simulink model "new_model_like_me"  (R2023a)
settings: Solver=FixedStepDiscrete  StartTime=0.0  StopTime=5  FixedStep=Ts  RelTol=1e-3  EnableMultiTasking=on
PreLoadFcn:
  | parameters_for_model_inn;
StopFcn:
  | ee_addSimlogTimeStamp(bdroot)
values from neighbouring files (symbols this model uses):
  deg = 10    [parameters_for_model_inn.m]
  Jm = 0.001368    [parameters_for_model_inn.m]
  Kaw_omega = 1    [parameters_for_model_inn.m]
  Ki_id = 3    [parameters_for_model_inn.m]
  Ki_iq = 20    [parameters_for_model_inn.m]
  Ki_omega = 2.2    [parameters_for_model_inn.m]
  Kp_id = 0.01    [parameters_for_model_inn.m]
  Kp_iq = 1.8    [parameters_for_model_inn.m]
  Kp_omega = 0.6    [parameters_for_model_inn.m]
  Kp_pos = 0.8    [parameters_for_model_inn.m]
  Ld = 0.00595    [parameters_for_model_inn.m]
  LimA2down = -80    [parameters_for_model_inn.m]
  LimA2up = 64    [parameters_for_model_inn.m]
  Lq = 0.00595    [parameters_for_model_inn.m]
  p = 4    [parameters_for_model_inn.m]
  psim = 0.180694733685904    (= 0.180694733686)    [parameters_for_model_inn.m]
  Red = 34.68    [parameters_for_model_inn.m]
  Tid_start = Tiq_stop + 0.02    (= 0.1)    [parameters_for_model_inn.m]
  Tid_stop = Tid_start + 0.04    (= 0.14)    [parameters_for_model_inn.m]
  Tiq_start = 0.02    [parameters_for_model_inn.m]
  Tiq_stop = Tiq_start + 0.06    (= 0.08)    [parameters_for_model_inn.m]
  Tomega_start = Tid_stop + 0.02    (= 0.16)    [parameters_for_model_inn.m]
  Tomega_stop = Tomega_start + 0.06    (= 0.22)    [parameters_for_model_inn.m]
  Tpos_start = Tomega_stop + 0.02    (= 0.24)    [parameters_for_model_inn.m]
  Tpos_stop = Tpos_start + 0.06    (= 0.3)    [parameters_for_model_inn.m]
  Ts = 5e-5    (= 5e-05)    [parameters_for_model_inn.m]
  Tsi = Ts * 20    (= 0.001)    [parameters_for_model_inn.m]
  Tso = Ts * 200    (= 0.01)    [parameters_for_model_inn.m]
  V1 = 250    [parameters_for_model_inn.m]
  Vnom = 300    [parameters_for_model_inn.m]
  Wmax = 7000    [parameters_for_model_inn.m]
  Wnom = 1800    [parameters_for_model_inn.m]
undefined symbols (not defined in the file or in its folder): DiscIntNeverNeededParam, Kd_pos, Ki_pos, Kn_pos, Tpos, X, Y, Z
libraries: nesl_utility x18, fl_lib x10, sm_lib x8, slctrlblks x6, ee_lib x5, eeTransforms x3, dspfdesign x3, eePmsmCurrentController x2, simulink x2, slpidlib x2, robotmaniplib x2, batteryecm_lib x1
(part 1 of 2)
CloseFcn:
  | try,close(h1_ee_ipmsm_velocity_control),end
  | clear h1_ee_ipmsm_velocity_control
  | 
  | clear simlog_ee_ipmsm_velocity_control
  | clear logsout_ee_ipmsm_velocity_control
  | 
  | clear Pmax Tmax p psim Ld Lq L0 Rs Jm Imax Wmax ans RT_Time RedTrq Red
  | clear Cdc Vnom V1 AH0
  | clear Ts fsw Tpos Tsi Tso Kp_id Ki_id Kp_iq Ki_iq Clock_fcn fn
  | clear numd_id dend_id numd_iq dend_iq psim
  | clear Kp_omega Ki_omega Kn_omega numd_omega dend_omega Kp_pos Ki_pos Kn_pos Kd_pos
  | clear ID_MAP IQ_MAP RPM_VECT TQ_VECT VDC_VECT
  | clear Link2 ArmInfo tout
Description:
  | IPMSM Full Control
settings Model: PauseTimes=0  Creator=KolobovBK  LastModifiedBy=kolobov_bk
settings SolverCC: AlgebraicLoopSolver=TrustRegion  AutoInsertRateTranBlk=on  MaxZcPerStep=1
settings DataIOCC: MaxDataPoints=210000  DSMLogging=off  ReturnWorkspaceOutputs=off  SignalLoggingName=logsout_ee_ipmsm_velocity_control
settings OptimizationCC: ReuseModelBlockBuffer=off  LifeSpan=inf
settings DebuggingCC: UnderspecifiedInitializationDetection=Classic  MergeDetectMultiDrivingBlocksExec=none  UnconnectedInputMsg=warning  UnconnectedOutputMsg=warning  UnconnectedLineMsg=warning  SFUnexpectedBacktrackingDiag=warning  SFNoUnconditionalDefaultTransitionDiag=warning  SFExecutionAtInitializationDiag=none  ArithmeticOperatorsInVariantConditions=warning
settings ModelReferenceCC: EnableRefExpFcnMdlSchedulingChecks=on
settings SFSimCC: SimUseLocalCustomCode=off  CustomCodeUndefinedFunction=UseInterfaceOnly
settings RTWCC: RTWUseLocalCustomCode=off  DLArmComputeVersion=19.05
settings CodeAppCC: StateflowObjectComments=on
settings GRTTargetCC: TargetLangStandard=C89/C90 (ANSI)
settings ConfigComp: CovMetricSettings=dw  CovSaveCumulativeToWorkspaceVar=on  CovSaveSingleToWorkspaceVar=on  CovExternalEMLEnable=off
settings SimscapeCC: SimscapeNormalizeSystem=off  SimscapeLogType=all  SimscapeLogSimulationStatistics=on  SimscapeLogName=simlog_ee_ipmsm_velocity_control  SimscapeLogDataHistory=210000

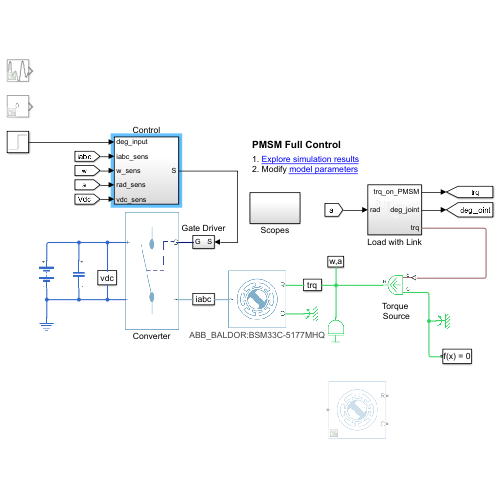
[thumbnail: Simulink's stored preview of the top-level diagram]
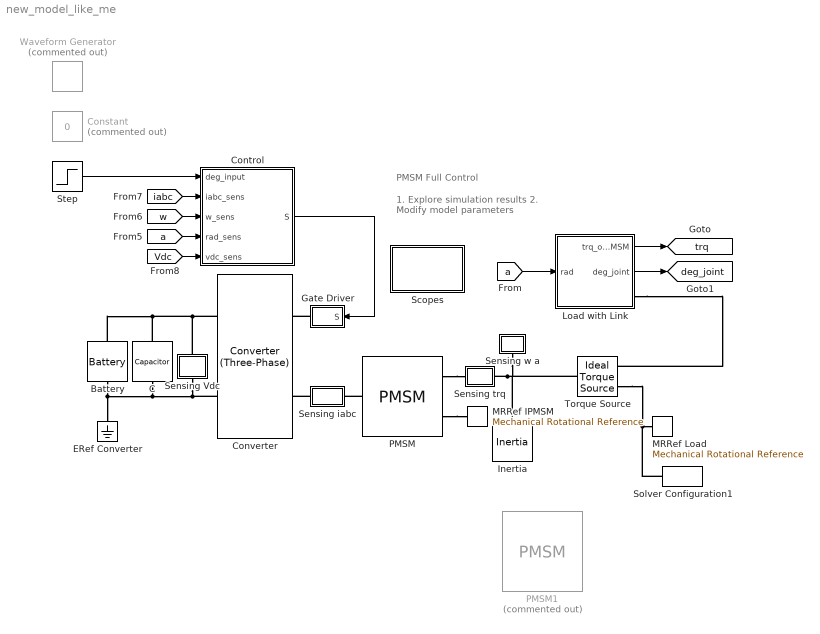
== system new_model_like_me ==
  note: PMSM Full Control
  note: 1. Explore simulation results
      | 2. Modify model parameters
  Battery : batteryecm_lib/Battery  Vnom=Vnom V  prm_dir=1  R1_dis=2 Ohm  R1_ch=2 Ohm  R1=0.001 Ohm  prm_AH=1  AH=300 hr*A  V1=V1 V  AH1=100 hr*A  prm_R2=1  R2=2000 Ohm  Tmeas=298.15 K  charge_measurement_port=simscape.enum.battery.enable.no  prm_dyn=1  Rp1=0.005 Ohm  tau1=30 s  Rp2=0.005 Ohm  tau2=30 s  Rp3=0.005 Ohm  tau3=30 s  Rp4=0.005 Ohm  tau4=30 s  Rp5=0.005 Ohm  tau5=30 s  prm_fade=1  N_fade=100  AH_fade=45 hr*A  R1_fade=2.02 Ohm  R1_ch_fade=2.02 Ohm  V1_fade=10.35 V  prm_age=1  prm_age_OCV=1  OCV_age=0.9  SOC_age=60  Tmeas_age=298.15 K  delta_time_age_vec=[0] d  temperature_age_vec=[273] K  OCV_scaling_age=2.2134e6  OCV_offset_age=1.632e6  temp_exp_age=0.515833569 V  t_exp_age=0.75  Vnom_T2=12 V  R1_T2=2.2 Ohm  R1_T2_dis=2.2 Ohm  R1_T2_ch=2.2 Ohm  V1_T2=11.4 V  R2_T2=2200 Ohm  Rp1_T2=0.005 Ohm  tau1_T2=30 s  Rp2_T2=0.005 Ohm  tau2_T2=30 s  Rp3_T2=0.005 Ohm  tau3_T2=30 s  Rp4_T2=0.005 Ohm  tau4_T2=30 s  Rp5_T2=0.005 Ohm  tau5_T2=30 s  Tmeas2=273.15 K  thermal_port=simscape.enum.thermaleffects.omit  thermal_mass=30000 J/K  i_specify=off  i_priority=None  i=0 A  i_nominal_specify=off  i_nominal_unit=A  i_nominal_value=1  v_specify=on  v_priority=High  v=300 V  v_nominal_specify=off  v_nominal_unit=V  v_nominal_value=1  charge_specify=on  charge_priority=High  charge=AH0 hr*A  charge_nominal_specify=off  charge_nominal_unit=A*hr  charge_nominal_value=1  num_cycles_specify=off  num_cycles_priority=High  num_cycles=0  num_cycles_nominal_specify=off  num_cycles_nominal_unit=1  num_cycles_nominal_value=1  temperature_specify=off  temperature_priority=High  temperature=298.15 K  temperature_nominal_specify=off  temperature_nominal_unit=K  temperature_nominal_value=1
  C : fl_lib/Electrical/Electrical Elements/Capacitor  c=Cdc F  r=1e-6 Ohm  g=0 1/Ohm  i_specify=off  i_priority=None  i=0 A  i_nominal_specify=off  i_nominal_unit=A  i_nominal_value=1  v_specify=off  v_priority=None  v=0 V  v_nominal_specify=off  v_nominal_unit=V  v_nominal_value=1  vc_specify=on  vc_priority=None  vc=Vnom V  vc_nominal_specify=off  vc_nominal_unit=V  vc_nominal_value=1
  Constant : Constant  Commented=on  Value=0
  Control : Subsystem
  Converter : ee_lib/Semiconductors & Converters/Converters/Converter (Three-Phase)  port_option=ee.enum.threePhasePort.composite  device_type=3  K=0  Vf=0.8 V  Ron=0.001 Ohm  Rds=0.001 Ohm  Goff=1e-5 1/Ohm  Vgt=1 V  Vgt_off=-1 V  Ih=1 A  Vth=0.5 V  diode_param=2  diode_Vf=0.8 V  diode_Ron=0.001 Ohm  diode_Goff=1e-5 1/Ohm  diode_C=50 nF  diode_iRM=-235 A  diode_iF=300 A  diode_idot=-50 A/us  diode_trr_param=1  diode_trr_factor=3  diode_trr=15 us  diode_Qrr=1.5e+3 s*uA  snubber_type=0  Cs=1e-7 F  Rs=0.1 Ohm
  ERef Converter : fl_lib/Electrical/Electrical Elements/Electrical Reference
  Gate Driver : Subsystem
  Inertia : fl_lib/Mechanical/Rotational Elements/Inertia  inertia=Jm kg*m^2  num_ports=foundation.enum.numPorts2.one  w_specify=on  w_priority=High  w=0 rpm  w_nominal_specify=off  w_nominal_unit=rad/s  w_nominal_value=1  t_specify=off  t_priority=High  t=0 N*m  t_nominal_specify=off  t_nominal_unit=N*m  t_nominal_value=1
  Load with Link : Subsystem
  MRRef IPMSM : fl_lib/Mechanical/Rotational Elements/Mechanical Rotational Reference
  MRRef Load : fl_lib/Mechanical/Rotational Elements/Mechanical Rotational Reference
  PMSM : ee_lib/Electromechanical/Permanent Magnet/PMSM  Tag={'toolbox/physmod/elec/library/m/ee_lib_parts';'Electromechanical/Permanent_Magnet/PMSM/ABB_BALDOR/BSM33C_5177MHQ.xml'}  port_option=ee.enum.threePhasePort.composite  winding_type=ee.enum.statorconnection.wye  machine_param=ee.enum.pmsm.parameterization.constant  nPolePairs=4  pmflux_param=ee.enum.pmflux.fluxlinkage  pm_flux_linkage=0.180694733685904 Wb  torque_constant=0.722778934743618 N*m/A  back_emf_constant=0.722778934743618 V/(rad/s)  stator_param=ee.enum.statorparam.LdLqL0  Ld=0.00595 H  Lq=0.00595 H  idVec=[-200 0 200] % Parameter not set A  iqVec=[-200 0 200] % Parameter not set A  LdMatrix=[0.0002 0.0002 0.0002;0.0002 0.0002 0.0002;0.0002 0.0002 0.0002] % Parameter not set H  LqMatrix=[0.0002 0.0002 0.0002;0.0002 0.0002 0.0002;0.0002 0.0002 0.0002] % Parameter not set H  PmMatrix=[0.1 0.1 0.1;0.1 0.1 0.1;0.1 0.1 0.1] Wb  ktMatrix=[0.18 0.18 0.18;0.18 0.18 0.18;0.18 0.18 0.18] N*m/A  keMatrix=[0.18 0.18 0.18;0.18 0.18 0.18;0.18 0.18 0.18] % Parameter not set V/(rad/s)  L0=[] % Parameter not set H  Ls=0.0002 H  Lm=-2e-05 H  Ms=2e-05 H  Rs=1.02 Ohm  zero_sequence=ee.enum.park.zerosequence.exclude  axes_param=ee.enum.rotorangle.daxis  loss_param=ee.enum.ironloss.none  losses_oc=[0 0 0] % Parameter not set W  losses_sc=[0 0 0] % Parameter not set W  f_losses=60 % Parameter not set Hz  Isc_losses=95 % Parameter not set A  J=0.001368 kg*m^2  lam=0 % Parameter not set N*m/(rad/s)  i_d_specify=off  i_d_priority=None  i_d=0 A  i_d_nominal_specify=off  i_d_nominal_unit=A  i_d_nominal_value=1  i_q_specify=off  i_q_priority=None  i_q=0 A  i_q_nominal_specify=off  i_q_nominal_unit=A  i_q_nominal_value=1  torque_specify=off  torque_priority=None  torque=0 N*m  torque_nominal_specify=off  torque_nominal_unit=N*m  torque_nominal_value=1  angular_velocity_specify=on  angular_velocity_priority=High  angular_velocity=0 rpm  angular_velocity_nominal_specify=off  angular_velocity_nominal_unit=rpm  angular_velocity_nominal_value=1  angular_position_specify=on  angular_position_priority=High  angular_position=0 deg  angular_position_nominal_specify=off  angular_position_nominal_unit=deg  angular_position_nominal_value=1  alpha=3.93e-3 1/K  alpha_flux=-0.001 1/K  Tmeas=298.15 K  stator_thermal_mass=100 J/K  rotor_thermal_mass=200 J/K  Rm_percent_rotor=90  Rd_percent_rotor=30  temperatureA_specify=off  temperatureA_priority=High  temperatureA=25 degC  temperatureA_nominal_specify=off  temperatureA_nominal_unit=degC  temperatureA_nominal_value=1  temperatureB_specify=off  temperatureB_priority=High  temperatureB=25 degC  temperatureB_nominal_specify=off  temperatureB_nominal_unit=degC  temperatureB_nominal_value=1  temperatureC_specify=off  temperatureC_priority=High  temperatureC=25 degC  temperatureC_nominal_specify=off  temperatureC_nominal_unit=degC  temperatureC_nominal_value=1  temperatureR_specify=off  temperatureR_priority=High  temperatureR=25 degC  temperatureR_nominal_specify=off  temperatureR_nominal_unit=degC  temperatureR_nominal_value=1
      settings: AttributesFormatString=ABB_BALDOR:BSM33C-5177MHQ  InternalSimscapePortConfiguration="{\"Bottom\":[],\"Left\":[{\"id\":\"N\",\"label\":\"~\",\"type\":\"foundation.electrical.three_phase\"}],\"Right\":[{\"id\":\"R\",\"label\":\"R\",\"type\":\"foundation.mechanical.rotational.rotational\"},{\"id\":\"C\",\"label\":\"C\",\"type\":\"foundation.mechanical.rotational.rotational\"}],\"Top\":[]}"
  PMSM1 : ee_lib/Electromechanical/Permanent Magnet/PMSM  Commented=on  port_option=ee.enum.threePhasePort.composite  winding_type=ee.enum.statorconnection.wye  machine_param=ee.enum.pmsm.parameterization.constant  nPolePairs=p  pmflux_param=ee.enum.pmflux.fluxlinkage  pm_flux_linkage=psim Wb  torque_constant=0.93 N*m/A  back_emf_constant=0.722778934743618 V/(rad/s)  stator_param=ee.enum.statorparam.LdLqL0  Ld=Ld H  Lq=Lq H  idVec=[-200 0 200] % Parameter not set A  iqVec=[-200 0 200] % Parameter not set A  LdMatrix=[0.0002 0.0002 0.0002;0.0002 0.0002 0.0002;0.0002 0.0002 0.0002] % Parameter not set H  LqMatrix=[0.0002 0.0002 0.0002;0.0002 0.0002 0.0002;0.0002 0.0002 0.0002] % Parameter not set H  PmMatrix=[0.1 0.1 0.1;0.1 0.1 0.1;0.1 0.1 0.1] Wb  ktMatrix=[0.18 0.18 0.18;0.18 0.18 0.18;0.18 0.18 0.18] N*m/A  keMatrix=[0.18 0.18 0.18;0.18 0.18 0.18;0.18 0.18 0.18] % Parameter not set V/(rad/s)  L0=L0 H  Ls=0.0002 H  Lm=-2e-05 H  Ms=2e-05 H  Rs=Rs Ohm  zero_sequence=ee.enum.park.zerosequence.exclude  axes_param=ee.enum.rotorangle.qaxis  loss_param=ee.enum.ironloss.none  losses_oc=[0 0 0] % Parameter not set W  losses_sc=[0 0 0] % Parameter not set W  f_losses=60 % Parameter not set Hz  Isc_losses=95 % Parameter not set A  J=Jm kg*m^2  lam=0 % Parameter not set N*m/(rad/s)  i_d_specify=off  i_d_priority=None  i_d=0 A  i_d_nominal_specify=off  i_d_nominal_unit=A  i_d_nominal_value=1  i_q_specify=off  i_q_priority=None  i_q=0 A  i_q_nominal_specify=off  i_q_nominal_unit=A  i_q_nominal_value=1  torque_specify=off  torque_priority=None  torque=0 N*m  torque_nominal_specify=off  torque_nominal_unit=N*m  torque_nominal_value=1  angular_velocity_specify=on  angular_velocity_priority=High  angular_velocity=0 rpm  angular_velocity_nominal_specify=off  angular_velocity_nominal_unit=rpm  angular_velocity_nominal_value=1  angular_position_specify=on  angular_position_priority=High  angular_position=0 deg  angular_position_nominal_specify=off  angular_position_nominal_unit=deg  angular_position_nominal_value=1  alpha=3.93e-3 1/K  alpha_flux=-0.001 1/K  Tmeas=298.15 K  stator_thermal_mass=100 J/K  rotor_thermal_mass=200 J/K  Rm_percent_rotor=90  Rd_percent_rotor=30  temperatureA_specify=off  temperatureA_priority=High  temperatureA=25 degC  temperatureA_nominal_specify=off  temperatureA_nominal_unit=degC  temperatureA_nominal_value=1  temperatureB_specify=off  temperatureB_priority=High  temperatureB=25 degC  temperatureB_nominal_specify=off  temperatureB_nominal_unit=degC  temperatureB_nominal_value=1  temperatureC_specify=off  temperatureC_priority=High  temperatureC=25 degC  temperatureC_nominal_specify=off  temperatureC_nominal_unit=degC  temperatureC_nominal_value=1  temperatureR_specify=off  temperatureR_priority=High  temperatureR=25 degC  temperatureR_nominal_specify=off  temperatureR_nominal_unit=degC  temperatureR_nominal_value=1
      settings: InternalSimscapePortConfiguration="{\"Bottom\":[],\"Left\":[{\"id\":\"N\",\"label\":\"~\",\"type\":\"foundation.electrical.three_phase\"}],\"Right\":[{\"id\":\"R\",\"label\":\"R\",\"type\":\"foundation.mechanical.rotational.rotational\"},{\"id\":\"C\",\"label\":\"C\",\"type\":\"foundation.mechanical.rotational.rotational\"}],\"Top\":[]}"
  Scopes : Subsystem
  Sensing Vdc : Subsystem
      mask Display: disp('vdc')
  Sensing trq : Subsystem
      mask Display: disp('trq')
  Sensing w a : Subsystem
      mask Display: disp('w,a')
  Sensing iabc : Subsystem
      mask Display: disp('iabc')
  Solver Configuration1 : nesl_utility/Solver Configuration  PhysicalDomain=network_engine_domain  SubClassName=solver  LeftPortType=input  RightPortType=generic  Tones=[]  Harmonics=[]  SimulateNoise=off  Profile=off  UseLocalSampling=off  EnableSwitchedLinearOptims=on  FrequencyDomain=off  UseCCode=off  RelTol=0.001  AbsTol=1e-06  MinStep=1e-09  ToWorkspace=off  RevertToSquareIcSolve=off  NumHomotopyIterations=100  PhasorMode=off  PhasorModeNumHarmonics=1  ConsistencySolver=NEWTON_FTOL  IndexReductionMethod=DerivativeReplacement  DoDC=off  ResidualTolerance=1e-9  ConsistencyTolSource=GLOBAL  ConsistencyAbsTol=0.001  ConsistencyRelTol=0.001  ConsistencyTolFactor=0.001  UseLocalSolver=on  LocalSolverChoice=NE_BACKWARD_EULER_ADVANCER  ResolveIndetEquations=on  FunctionEvalNumThread=1  LocalSolverSampleTime=Ts  DoFixedCost=on  MaxNonlinIter=5  MaxModeIter=2  ComputeImpulses=off  ImpulseIterations=2  LinearAlgebra=auto  LinearAlgebraNumThread=0  EquationFormulation=NE_TIME_EF  DelaysMemoryBudget=1024  AutomaticFiltering=on  FilteringTimeConstant=0.001  PartitionStorageMethod=AS_NEEDED  PartitionMemoryBudget=1024  PartitionMethod=FAST
  Step : Step  Time=0.5  After=deg  SampleTime=0
  Torque Source : fl_lib/Mechanical/Mechanical Sources/Ideal Torque Source
  Waveform Generator : simulink/Sources/Waveform Generator  Commented=on  OutMin=[]  OutMax=[]  OutDataTypeStr=double  SelectedSignal=1  Signals=sin(50, 3, 1)  BlockNames=MultiportSwitch_926a5b7303e4405  SampleTime=0.1
  tag scope: deg_joint=global, trq=global
  wires:
  Control/1(S) -> Gate Driver/1(S)
  [Vdc] -> Control/5(vdc_sens)
  [iabc] -> Control/2(iabc_sens)
  [w] -> Control/3(w_sens)
  [a] -> Control/4(rad_sens)
  [a] -> Load with Link/1(rad)
  Step/1 -> Control/1(deg_input)
  Load with Link/1(trq_on_PMSM) -> [trq]
  Load with Link/2(deg_joint) -> [deg_joint]
  connections:
  Converter/RConn1 -- Sensing Vdc/LConn1 -- Battery/LConn1 -- C/LConn1
  Sensing trq/RConn1 -- Inertia/LConn1 -- Torque Source/LConn1 -- Sensing w a/LConn1
  Gate Driver/RConn1 -- Converter/LConn1
  Torque Source/RConn2 -- Solver Configuration1/RConn1 -- MRRef Load/LConn1
  Sensing iabc/LConn1 -- Converter/LConn2
  Battery/RConn1 -- Converter/RConn2 -- Sensing Vdc/RConn1 -- C/RConn1 -- ERef Converter/LConn1
  PMSM/LConn1 -- Sensing iabc/RConn1
  PMSM/RConn1 -- Sensing trq/LConn1
  PMSM/RConn2 -- MRRef IPMSM/LConn1
  Load with Link/RConn1 -- Torque Source/RConn1

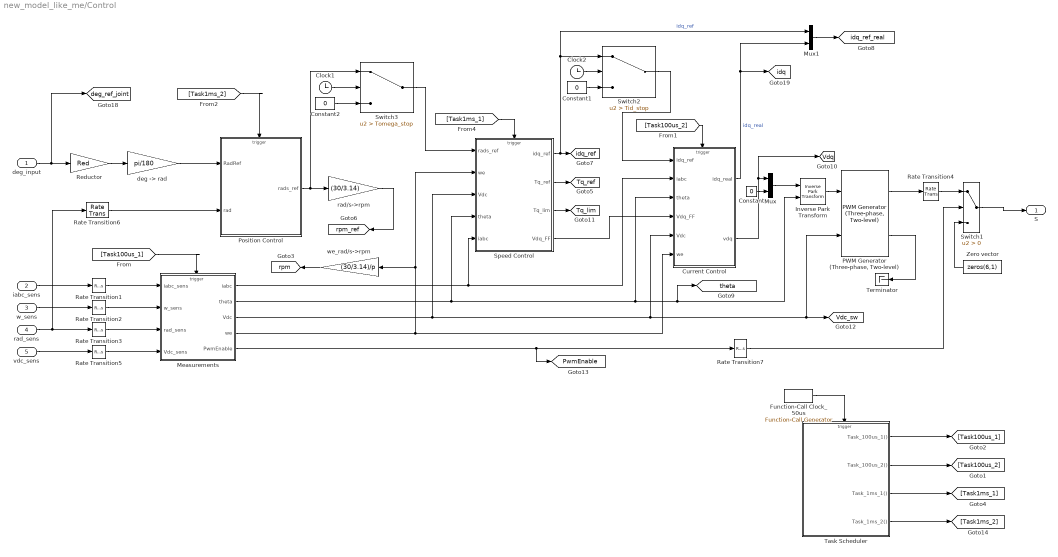
== system new_model_like_me/Control ==
  deg_input : Inport
  iabc_sens : Inport  Port=2
  w_sens : Inport  Port=3
  rad_sens : Inport  Port=4
  vdc_sens : Inport  Port=5
  Clock1 : Clock
  Clock2 : Clock
  Constant : Constant  Value=0  SampleTime=-1
  Constant1 : Constant  Value=0
  Constant2 : Constant  Value=0
  Current Control : Subsystem
  Function-Call Clock_50us : simulink/Ports & Subsystems/Function-Call Generator  sample_time=Clock_fcn  numberOfIterations=1  DisallowWideOutput=off
  Inverse Park Transform : eeTransforms/Inverse Park Transform  AxisAlignment=Q-axis  PowerInvariant=off
  Measurements : Subsystem
  Mux : Mux  Inputs=2
  Mux1 : Mux  Inputs=2
  "PWM Generator (Three-phase, Two-level)" : eePwmGeneratorTwoLevel/PWM Generator (Three-phase, Two-level)  PWMMode=Continuous PWM (CPWM)  CPWMMode=SVM: space vector modulation  DPWMMode=60 DPWM: 60 degree discontinuous PWM  fsw=fsw  Ts=Ts
  Position Control : Subsystem
  Rate Transition{1..7} (7 alike) : RateTransition
  Reductor : Gain  Gain=Red
  Speed Control : Subsystem
  Switch1 : Switch  Criteria=u2 > Threshold  SaturateOnIntegerOverflow=off  InputSameDT=off
  Switch2 : Switch  Criteria=u2 > Threshold  Threshold=Tid_stop  SaturateOnIntegerOverflow=off  InputSameDT=off
  Switch3 : Switch  Criteria=u2 > Threshold  Threshold=Tomega_stop  SaturateOnIntegerOverflow=off  InputSameDT=off
  Task Scheduler : Stateflow chart  TreatAsAtomicUnit=on
  Terminator : Terminator
  Zero vector : Constant  Value=zeros(6,1)
  "deg -> rad" : Gain  Gain=pi/180
  rad/s->rpm : Gain  Gain=(30/3.14)
  we_rad/s->rpm : Gain  Gain=(30/3.14)/p
  S : Outport  VectorParamsAs1DForOutWhenUnconnected=off
  tag scope: PwmEnable=global, Tq_lim=global, Tq_ref=global, Vdc_sw=global, Vdq=global, deg_ref_joint=global, idq=global, idq_ref=global, idq_ref_real=global, rpm=global, rpm_ref=global, theta=global
  wires:
  [Task100us_1] -> Measurements/Trigger
  [Task100us_2] -> Current Control/Trigger
  Current Control/2(vdq) -> Mux/1, [Vdq]
  Measurements/1(iabc) -> Current Control/2(iabc), Speed Control/5(iabc)
  Measurements/2(theta) -> Inverse Park Transform/2, [theta], Current Control/3(theta), Speed Control/4(theta)
  "PWM Generator (Three-phase, Two-level)"/1 -> Rate Transition4/1
  Inverse Park Transform/1 -> "PWM Generator (Three-phase, Two-level)"/1
  iabc_sens/1 -> Rate Transition1/1
  w_sens/1 -> Rate Transition2/1
  vdc_sens/1 -> Rate Transition5/1
  "PWM Generator (Three-phase, Two-level)"/2 -> Terminator/1
  Rate Transition1/1 -> Measurements/1(iabc_sens)
  Rate Transition2/1 -> Measurements/2(w_sens)
  Rate Transition3/1 -> Measurements/3(rad_sens)
  Rate Transition5/1 -> Measurements/4(Vdc_sens)
  Measurements/3(Vdc) -> [Vdc_sw], "PWM Generator (Three-phase, Two-level)"/2, Current Control/5(Vdc), Speed Control/3(Vdc)
  Speed Control/2(Tq_ref) -> [Tq_ref]
  Speed Control/3(Tq_lim) -> [Tq_lim]
  Switch1/1 -> S/1
  Rate Transition4/1 -> Switch1/1
  Measurements/5(PwmEnable) -> [PwmEnable], Rate Transition7/1
  Zero vector/1 -> Switch1/3
  Rate Transition7/1 -> Switch1/2
  [Task1ms_1] -> Speed Control/Trigger
  Mux/1 -> Inverse Park Transform/1
  Constant/1 -> Mux/2
  deg_input/1 -> [deg_ref_joint], Reductor/1
  Rate Transition6/1 -> Position Control/2(rad)
  Function-Call Clock_50us/1 -> Task Scheduler/Trigger
  Task Scheduler/1(Task_100us_1()) -> [Task100us_1]
  Task Scheduler/2(Task_100us_2()) -> [Task100us_2]
  Task Scheduler/3(Task_1ms_1()) -> [Task1ms_1]
  Measurements/4(we) -> Speed Control/2(we), we_rad/s->rpm/1, Current Control/6(we)
  we_rad/s->rpm/1 -> [rpm]
  rad/s->rpm/1 -> [rpm_ref]
  [Task1ms_2] -> Position Control/Trigger
  Task Scheduler/4(Task_1ms_2()) -> [Task1ms_2]
  Reductor/1 -> "deg -> rad"/1
  Speed Control/4(Vdq_FF) -> Current Control/4(Vdq_FF)
  "deg -> rad"/1 -> Position Control/1(RadRef)
  rad_sens/1 -> Rate Transition3/1, Rate Transition6/1
  Position Control/1(rads_ref) -> Switch3/1, rad/s->rpm/1
  Clock1/1 -> Switch3/2
  Constant2/1 -> Switch3/3
  Switch3/1 -> Speed Control/1(rads_ref)
  Speed Control/1(idq_ref) -> Mux1/1, Switch2/1, [idq_ref]  "idq_ref"
  Current Control/1(idq_real) -> [idq], Mux1/2  "idq_real"
  Mux1/1 -> [idq_ref_real]
  Clock2/1 -> Switch2/2
  Constant1/1 -> Switch2/3
  Switch2/1 -> Current Control/1(idq_ref)

== system new_model_like_me/Gate Driver ==
  S : Inport
  Demux : Demux  Outputs=6
  Simulink-PS Converter{1..6} (6 alike) : nesl_utility/Simulink-PS Converter  PhysicalDomain=network_engine_domain  SubClassName=ps_input  LeftPortType=input  RightPortType=output  PseudoPeriodic=off  Frequencies=[]  NoiseDistribution=none  NoiseParameters=[]  Unit=1  AffineConversion=off  FilteringAndDerivatives=zero  SimscapeFilterOrder=1  InputFilterTimeConstant=0.001  UdotUserProvided=1
  Six-Pulse Gate Multiplexer : ee_lib/Semiconductors & Converters/Converters/Six-Pulse Gate Multiplexer  port_option=ee.enum.controlport.ps
  G : PMIOPort  Side=Right
  wires:
  Demux/1 -> Simulink-PS Converter1/1
  S/1 -> Demux/1
  Demux/4 -> Simulink-PS Converter4/1
  Demux/2 -> Simulink-PS Converter2/1
  Demux/3 -> Simulink-PS Converter3/1
  Demux/5 -> Simulink-PS Converter5/1
  Demux/6 -> Simulink-PS Converter6/1
  connections:
  Six-Pulse Gate Multiplexer/RConn1 -- G/RConn1
  Simulink-PS Converter1/RConn1 -- Six-Pulse Gate Multiplexer/LConn1
  Simulink-PS Converter3/RConn1 -- Six-Pulse Gate Multiplexer/LConn3
  Simulink-PS Converter5/RConn1 -- Six-Pulse Gate Multiplexer/LConn5
  Simulink-PS Converter6/RConn1 -- Six-Pulse Gate Multiplexer/LConn6
  Simulink-PS Converter4/RConn1 -- Six-Pulse Gate Multiplexer/LConn4
  Simulink-PS Converter2/RConn1 -- Six-Pulse Gate Multiplexer/LConn2

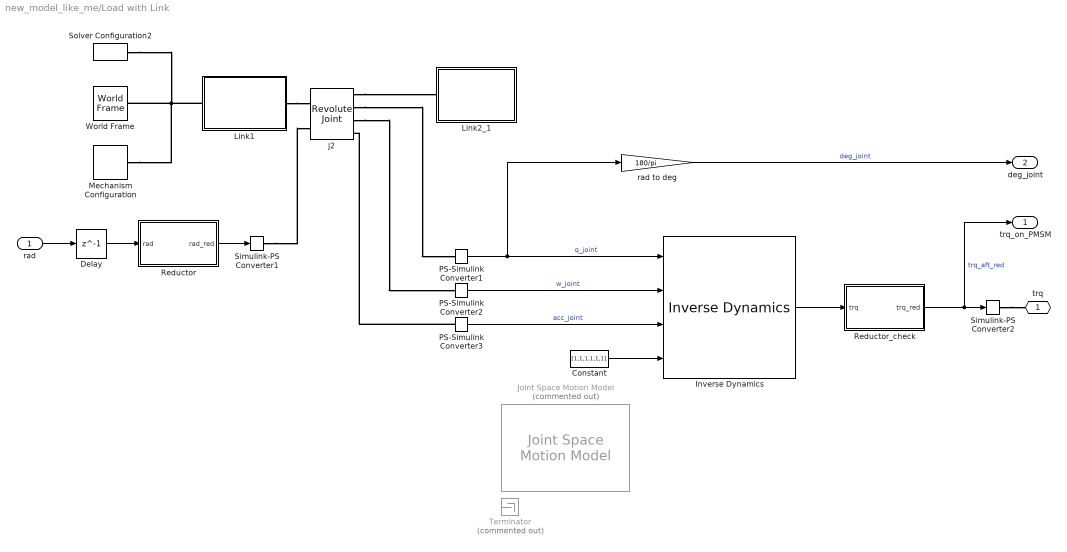
== system new_model_like_me/Load with Link ==
  rad : Inport
  Constant : Constant  Value=[1,1,1,1,1,1]
  Delay : Delay  DelayLength=1
  Inverse Dynamics : robotmaniplib/Inverse Dynamics  RigidBodyTree=Link2  SimulateUsing=Interpreted execution
  Joint Space Motion Model : robotmaniplib/Joint Space Motion Model  Commented=on  RigidBodyTree=Link2  MotionType=PD Control  ProportionalGain=100  DerivativeGain=10  ErrorDynamicsSpecification=Step Response  DampingRatio=0.45595  NaturalFrequency=877.2895  SettlingTime=0.01  Overshoot=0.2  ShowExternalForcePort=off  InitConfig=0  InitJointVel=0  SimulateUsing=Interpreted execution
  Link1 : Subsystem
  Link2_1 : Subsystem
  Mechanism Configuration : sm_lib/Utilities/Mechanism Configuration  UniformGravity=Constant  GravityVector=[0 0 -9.80665]  GravityVectorUnits=m/s^2  LinearizationDelta=0.001  JointModeTransitionNonlinearIterations=2
  PS-Simulink Converter1 : nesl_utility/PS-Simulink Converter  PhysicalDomain=network_engine_domain  SubClassName=ps_output  LeftPortType=input  RightPortType=output  PseudoPeriodic=off  Frequencies=[]  VectorFormat=inherit  Unit=inherit  AffineConversion=off
  PS-Simulink Converter2 : nesl_utility/PS-Simulink Converter  PhysicalDomain=network_engine_domain  SubClassName=ps_output  LeftPortType=input  RightPortType=output  PseudoPeriodic=off  Frequencies=[]  VectorFormat=inherit  Unit=inherit  AffineConversion=off
  PS-Simulink Converter3 : nesl_utility/PS-Simulink Converter  PhysicalDomain=network_engine_domain  SubClassName=ps_output  LeftPortType=input  RightPortType=output  PseudoPeriodic=off  Frequencies=[]  VectorFormat=inherit  Unit=inherit  AffineConversion=off
  Reductor : Subsystem
  Reductor_check : Subsystem
  Simulink-PS Converter1 : nesl_utility/Simulink-PS Converter  PhysicalDomain=network_engine_domain  SubClassName=ps_input  LeftPortType=input  RightPortType=output  PseudoPeriodic=off  Frequencies=[]  NoiseDistribution=none  NoiseParameters=[]  Unit=rad  AffineConversion=off  FilteringAndDerivatives=zero  SimscapeFilterOrder=1  InputFilterTimeConstant=0.001  UdotUserProvided=0
  Simulink-PS Converter2 : nesl_utility/Simulink-PS Converter  PhysicalDomain=network_engine_domain  SubClassName=ps_input  LeftPortType=input  RightPortType=output  PseudoPeriodic=off  Frequencies=[]  NoiseDistribution=none  NoiseParameters=[]  Unit=N*m  AffineConversion=off  FilteringAndDerivatives=provide  SimscapeFilterOrder=1  InputFilterTimeConstant=0.001  UdotUserProvided=0
  Solver Configuration2 : nesl_utility/Solver Configuration  PhysicalDomain=network_engine_domain  SubClassName=solver  LeftPortType=input  RightPortType=generic  Tones=[]  Harmonics=[]  SimulateNoise=off  Profile=off  UseLocalSampling=off  EnableSwitchedLinearOptims=on  FrequencyDomain=off  UseCCode=off  RelTol=0.001  AbsTol=1e-06  MinStep=1e-09  ToWorkspace=off  RevertToSquareIcSolve=off  NumHomotopyIterations=100  PhasorMode=off  PhasorModeNumHarmonics=1  ConsistencySolver=NEWTON_FTOL  IndexReductionMethod=DerivativeReplacement  DoDC=off  ResidualTolerance=1e-9  ConsistencyTolSource=GLOBAL  ConsistencyAbsTol=0.001  ConsistencyRelTol=0.001  ConsistencyTolFactor=0.001  UseLocalSolver=on  LocalSolverChoice=NE_BACKWARD_EULER_ADVANCER  ResolveIndetEquations=on  FunctionEvalNumThread=1  LocalSolverSampleTime=Ts  DoFixedCost=on  MaxNonlinIter=5  MaxModeIter=2  ComputeImpulses=off  ImpulseIterations=2  LinearAlgebra=auto  LinearAlgebraNumThread=0  EquationFormulation=NE_TIME_EF  DelaysMemoryBudget=1024  AutomaticFiltering=on  FilteringTimeConstant=0.001  PartitionStorageMethod=AS_NEEDED  PartitionMemoryBudget=1024  PartitionMethod=FAST
  Terminator : Terminator  Commented=on
  World Frame : sm_lib/Frames and Transforms/World Frame
  j2 : sm_lib/Joints/Revolute Joint  JointMode=Normal  SenseConstraintForce=off  SenseConstraintForceX=off  SenseConstraintForceY=off  SenseConstraintForceZ=off  SenseConstraintTorque=off  SenseConstraintTorqueX=off  SenseConstraintTorqueY=off  SenseConstraintTorqueZ=off  SenseTotalForce=off  SenseTotalForceX=off  SenseTotalForceY=off  SenseTotalForceZ=off  SenseTotalTorque=off  SenseTotalTorqueX=off  SenseTotalTorqueY=off  SenseTotalTorqueZ=off  CompositeWrenchDir=FollowerOnBase  CompositeWrenchFrame=BaseFrame  EquilibriumPosition=0  EquilibriumPositionUnits=deg  SpringStiffness=4.92  SpringStiffnessUnits=N*m/deg  DampingCoefficient=0  DampingCoefficientUnits=N*m/(deg/s)  TorqueActuationMode=ComputedTorque  MotionActuationMode=InputMotion  SensePosition=on  SenseVelocity=on  SenseAcceleration=on  SenseTorqueForce=off  SenseLowerLimitTorqueForce=off  SenseUpperLimitTorqueForce=off  LowerLimitSpecify=on  LowerLimitBound=-120  LowerLimitBoundUnits=deg  LowerLimitStiffness=1e4  LowerLimitStiffnessUnits=N*m/deg  LowerLimitDamping=10  LowerLimitDampingUnits=N*m/(deg/s)  LowerLimitTransitionRegionWidth=0.1  LowerLimitTransitionRegionWidthUnits=deg  UpperLimitSpecify=on  UpperLimitBound=120  UpperLimitBoundUnits=deg  UpperLimitStiffness=1e4  UpperLimitStiffnessUnits=N*m/deg  UpperLimitDamping=10  UpperLimitDampingUnits=N*m/(deg/s)  UpperLimitTransitionRegionWidth=0.1  UpperLimitTransitionRegionWidthUnits=deg  PositionTargetSpecify=off  PositionTargetPriority=High  PositionTargetValue=0  PositionTargetValueUnits=deg  VelocityTargetSpecify=off  VelocityTargetPriority=High  VelocityTargetValue=0  VelocityTargetValueUnits=deg/s
  rad to deg : Gain  Gain=180/pi
  trq : PMIOPort  Side=Right
  trq_on_PMSM : Outport
  deg_joint : Outport  Port=2
  wires:
  Reductor/1(rad_red) -> Simulink-PS Converter1/1
  PS-Simulink Converter1/1 -> rad to deg/1, Inverse Dynamics/1  "q_joint"
  PS-Simulink Converter2/1 -> Inverse Dynamics/2  "w_joint"
  rad/1 -> Delay/1
  Constant/1 -> Inverse Dynamics/4
  Delay/1 -> Reductor/1(rad)
  Inverse Dynamics/1 -> Reductor_check/1(trq)
  PS-Simulink Converter3/1 -> Inverse Dynamics/3  "acc_joint"
  Reductor_check/1(trq_red) -> trq_on_PMSM/1, Simulink-PS Converter2/1  "trq_aft_red"
  rad to deg/1 -> deg_joint/1  "deg_joint"
  connections:
  Simulink-PS Converter1/RConn1 -- j2/LConn2
  j2/RConn2 -- PS-Simulink Converter1/LConn1
  j2/RConn3 -- PS-Simulink Converter2/LConn1
  PS-Simulink Converter3/LConn1 -- j2/RConn4
  Simulink-PS Converter2/RConn1 -- trq/RConn1
  Mechanism Configuration/RConn1 -- Solver Configuration2/RConn1 -- World Frame/RConn1 -- Link1/LConn1
  j2/RConn1 -- Link2_1/LConn1
  Link1/RConn1 -- j2/LConn1

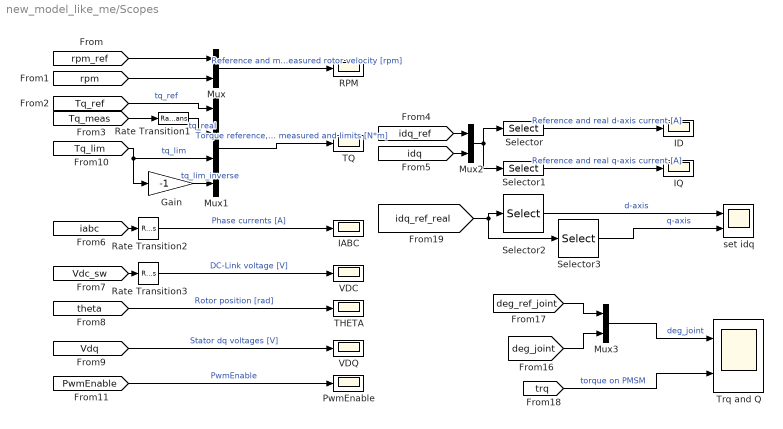
== system new_model_like_me/Scopes ==
  Gain : Gain  Gain=-1
  IABC : Scope
  ID : Scope
  IQ : Scope
  Mux : Mux  Inputs=2
  Mux1 : Mux
  Mux2 : Mux  Inputs=2
  Mux3 : Mux  Inputs=2
  PwmEnable : Scope
  RPM : Scope
  Rate Transition1 : RateTransition
  Rate Transition2 : RateTransition  OutPortSampleTime=RT_Time
  Rate Transition3 : RateTransition  OutPortSampleTime=RT_Time
  Selector : Selector  InputPortWidth=4  IndexOptions=Index vector (dialog)  Indices=[1 3]  OutputSizes=1
  Selector1 : Selector  InputPortWidth=4  IndexOptions=Index vector (dialog)  Indices=[2 4]  OutputSizes=1
  Selector2 : Selector  InputPortWidth=4  IndexOptions=Index vector (dialog)  Indices=[1 3]  OutputSizes=1
  Selector3 : Selector  InputPortWidth=4  IndexOptions=Index vector (dialog)  Indices=[2 4]  OutputSizes=1
  THETA : Scope
  TQ : Scope
  Trq and Q : Scope  NumInputPorts=2
  VDC : Scope
  VDQ : Scope
  set idq : Scope  NumInputPorts=2
  wires:
  [rpm] -> Mux/2
  Selector1/1 -> IQ/1  "Reference and real q-axis current [A]"
  Mux2/1 -> Selector1/1, Selector/1
  Gain/1 -> Mux1/4  "tq_lim_inverse"
  Rate Transition3/1 -> VDC/1  "DC-Link voltage [V]"
  [Vdc_sw] -> Rate Transition3/1
  [idq_ref] -> Mux2/1
  [PwmEnable] -> PwmEnable/1  "PwmEnable"
  Rate Transition2/1 -> IABC/1  "Phase currents [A]"
  [idq] -> Mux2/2
  [rpm_ref] -> Mux/1
  [iabc] -> Rate Transition2/1
  [Tq_meas] -> Rate Transition1/1
  [Vdq] -> VDQ/1  "Stator dq voltages [V]"
  Selector/1 -> ID/1  "Reference and real d-axis current [A]"
  [Tq_lim] -> Mux1/3, Gain/1  "tq_lim"
  Mux1/1 -> TQ/1  "Torque reference, measured and limits [N*m]"
  [theta] -> THETA/1  "Rotor position [rad]"
  Rate Transition1/1 -> Mux1/2  "tq_real"
  Mux/1 -> RPM/1  "Reference and measured rotor velocity [rpm]"
  [Tq_ref] -> Mux1/1  "tq_ref"
  [trq] -> Trq and Q/2  "torque on PMSM"
  Mux3/1 -> Trq and Q/1  "deg_joint"
  [deg_joint] -> Mux3/2
  [deg_ref_joint] -> Mux3/1
  Selector2/1 -> set idq/1  "d-axis"
  Selector3/1 -> set idq/2  "q-axis"
  [idq_ref_real] -> Selector3/1, Selector2/1

== system new_model_like_me/Sensing Vdc ==
  PS-Simulink Converter4 : nesl_utility/PS-Simulink Converter  PhysicalDomain=network_engine_domain  SubClassName=ps_output  LeftPortType=input  RightPortType=output  PseudoPeriodic=off  Frequencies=[]  VectorFormat=1-D array  Unit=V  AffineConversion=off
  Voltage Sensor : fl_lib/Electrical/Electrical Sensors/Voltage Sensor
  + : PMIOPort  Side=Left
  - : PMIOPort  Port=2  Side=Right
  tag scope: Vdc=global
  wires:
  PS-Simulink Converter4/1 -> [Vdc]
  connections:
  Voltage Sensor/LConn1 -- +/RConn1
  Voltage Sensor/RConn2 -- -/RConn1
  PS-Simulink Converter4/LConn1 -- Voltage Sensor/RConn1

== system new_model_like_me/Sensing trq ==
  PS-Simulink Converter3 : nesl_utility/PS-Simulink Converter  PhysicalDomain=network_engine_domain  SubClassName=ps_output  LeftPortType=input  RightPortType=output  PseudoPeriodic=off  Frequencies=[]  VectorFormat=1-D array  Unit=N*m  AffineConversion=off
  Torque Sensor : fl_lib/Mechanical/Mechanical Sensors/Ideal Torque Sensor
  R : PMIOPort  Side=Left
  C : PMIOPort  Port=2  Side=Right
  tag scope: Tq_meas=global
  wires:
  PS-Simulink Converter3/1 -> [Tq_meas]
  connections:
  Torque Sensor/RConn1 -- C/RConn1
  Torque Sensor/RConn2 -- PS-Simulink Converter3/LConn1
  Torque Sensor/LConn1 -- R/RConn1

== system new_model_like_me/Sensing w a ==
  MRRef : fl_lib/Mechanical/Rotational Elements/Mechanical Rotational Reference
  Motion Sensor : fl_lib/Mechanical/Mechanical Sensors/Ideal Rotational Motion Sensor  reference=foundation.enum.MeasurementReference.difference  acceleration_port=false  velocity_port=true  position_port=true  wrap_angle=false  offset=0 deg
  PS-Simulink Converter1 : nesl_utility/PS-Simulink Converter  PhysicalDomain=network_engine_domain  SubClassName=ps_output  LeftPortType=input  RightPortType=output  PseudoPeriodic=off  Frequencies=[]  VectorFormat=1-D array  Unit=rad/s  AffineConversion=off
  PS-Simulink Converter2 : nesl_utility/PS-Simulink Converter  PhysicalDomain=network_engine_domain  SubClassName=ps_output  LeftPortType=input  RightPortType=output  PseudoPeriodic=off  Frequencies=[]  VectorFormat=1-D array  Unit=rad  AffineConversion=off
  R : PMIOPort  Side=Left
  tag scope: a=global, w=global
  wires:
  PS-Simulink Converter1/1 -> [w]
  PS-Simulink Converter2/1 -> [a]
  connections:
  R/RConn1 -- Motion Sensor/LConn1
  Motion Sensor/RConn2 -- PS-Simulink Converter1/LConn1
  MRRef/LConn1 -- Motion Sensor/RConn1
  PS-Simulink Converter2/LConn1 -- Motion Sensor/RConn3

== system new_model_like_me/Sensing iabc ==
  Current Sensor : ee_lib/Sensors & Transducers/Current Sensor (Three-Phase)
  PS-Simulink Converter : nesl_utility/PS-Simulink Converter  PhysicalDomain=network_engine_domain  SubClassName=ps_output  LeftPortType=input  RightPortType=output  PseudoPeriodic=off  Frequencies=[]  VectorFormat=1-D array  Unit=A  AffineConversion=off
  1 : PMIOPort  Side=Left
  2 : PMIOPort  Port=2  Side=Right
  tag scope: iabc=global
  wires:
  PS-Simulink Converter/1 -> [iabc]
  connections:
  1/RConn1 -- Current Sensor/LConn1
  2/RConn1 -- Current Sensor/RConn2
  Current Sensor/RConn1 -- PS-Simulink Converter/LConn1

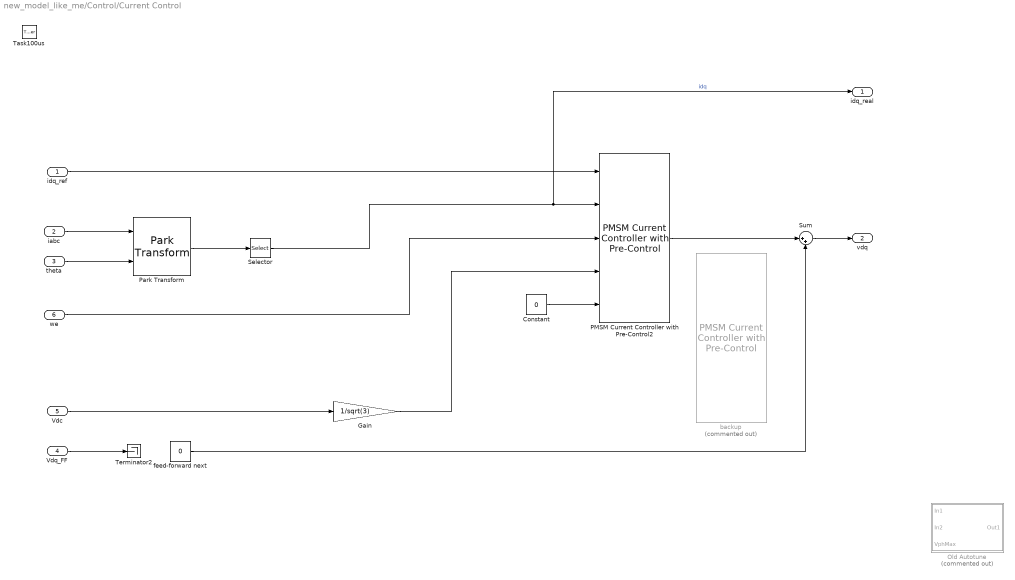
== system new_model_like_me/Control/Current Control ==
  idq_ref : Inport
  iabc : Inport  Port=2
  theta : Inport  Port=3
  Vdq_FF : Inport  Port=4
  Vdc : Inport  Port=5
  we : Inport  Port=6
  Task100us : TriggerPort  TriggerType=function-call  VariantControl=Variant  PortDimensions=1
  Constant : Constant  Value=0
  Gain : Gain  Gain=1/sqrt(3)
  Old Autotune : Subsystem  Commented=on
  PMSM Current Controller with Pre-Control2 : eePmsmCurrentController/PMSM Current Controller with Pre-Control  Kp_id=Kp_id  Ki_id=Ki_id  Kaw_id=Kaw_id  Kp_iq=Kp_iq  Ki_iq=Ki_iq  Kaw_iq=Kaw_iq  Ts=-1  Tsd=Ts  AxisPrio=Q-axis  ActZC=on  ActFF=on  idVect=[-200, 0, 200]  iqVect=[-200, 0, 200]  LdMatrix=Ld * ones(3, 3)  LqMatrix=Lq * ones(3, 3)  psimMatrix=psim * ones(3, 3)
  Park Transform : eeTransforms/Park Transform  AxisAlignment=Q-axis  PowerInvariant=off
  Selector : Selector  InputPortWidth=3  IndexOptions=Index vector (dialog)  Indices=[1 2]  OutputSizes=1
  Sum : Sum  Inputs=|++
  Terminator2 : Terminator
  backup : eePmsmCurrentController/PMSM Current Controller with Pre-Control  Commented=on  Kp_id=0.01  Ki_id=3  Kaw_id=1000  Kp_iq=2  Ki_iq=1500  Kaw_iq=50  Ts=-1  Tsd=Tsi  AxisPrio=Q-axis  ActZC=on  ActFF=off  idVect=[-200, 0, 200]  iqVect=[-200, 0, 200]  LdMatrix=Ld * ones(3, 3)  LqMatrix=Lq * ones(3, 3)  psimMatrix=psim * ones(3, 3)
  feed-forward next : Constant  Value=0
  idq_real : Outport
  vdq : Outport  Port=2  VectorParamsAs1DForOutWhenUnconnected=off
  wires:
  Park Transform/1 -> Selector/1
  Vdc/1 -> Gain/1
  Gain/1 -> PMSM Current Controller with Pre-Control2/4
  Selector/1 -> PMSM Current Controller with Pre-Control2/2, idq_real/1  "idq"
  idq_ref/1 -> PMSM Current Controller with Pre-Control2/1
  Sum/1 -> vdq/1
  Vdq_FF/1 -> Terminator2/1
  feed-forward next/1 -> Sum/2
  we/1 -> PMSM Current Controller with Pre-Control2/3
  Constant/1 -> PMSM Current Controller with Pre-Control2/5
  PMSM Current Controller with Pre-Control2/1 -> Sum/1
  iabc/1 -> Park Transform/1
  theta/1 -> Park Transform/2

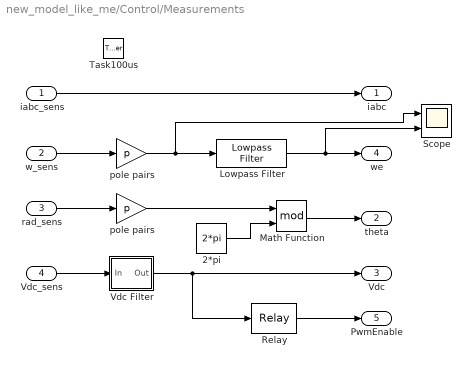
== system new_model_like_me/Control/Measurements ==
  iabc_sens : Inport
  w_sens : Inport  Port=2
  rad_sens : Inport  Port=3
  Vdc_sens : Inport  Port=4
  Task100us : TriggerPort  TriggerType=function-call  VariantControl=Variant  PortDimensions=1
  2*pi : Constant  Value=2*pi  SampleTime=-1
  Lowpass Filter : dspfdesign/Lowpass Filter  FilterType=FIR  DesignForMinimumOrder=on  FilterOrder=50  PassbandFrequency=2000  StopbandFrequency=5000  PassbandRipple=1  StopbandAttenuation=10  SampleRateMode=Specify on dialog  SampleRate=44000  SimulateUsing=Interpreted execution  roundingMode=Floor  coeffsDataTypeStr=fixdt(1,16)
  Math Function : Math  Operator=mod  SignedPower=on
  Relay : Relay  OnSwitchValue=V1  OffSwitchValue=0.5*V1
  Scope : Scope  NumInputPorts=2
  Vdc Filter : Subsystem  mask(Discrete first-order filter (Low-pass)){T=0.005, Ts=1e-4}
      mask prompts: T "Time constant (s):"; Ts "Sample time (s):"
      mask help: This block implements a discrete low-pass filter. To calculate the coefficients, the block discretises a continuous low-pass filter using the Tustin method.
      mask init:
      | num = [ Ts/(2*T + Ts), Ts/(2*T + Ts)];
      | den = [ 1, -(2*T - Ts)/(2*T + Ts)];
  pole pairs : Gain  Gain=p
  "pole pairs " : Gain  Gain=p
  iabc : Outport  VectorParamsAs1DForOutWhenUnconnected=off
  theta : Outport  Port=2  VectorParamsAs1DForOutWhenUnconnected=off
  Vdc : Outport  Port=3  VectorParamsAs1DForOutWhenUnconnected=off
  we : Outport  Port=4  VectorParamsAs1DForOutWhenUnconnected=off
  PwmEnable : Outport  Port=5  VectorParamsAs1DForOutWhenUnconnected=off
  wires:
  Vdc_sens/1 -> Vdc Filter/1(In)
  w_sens/1 -> pole pairs/1
  2*pi/1 -> Math Function/2
  Relay/1 -> PwmEnable/1
  Vdc Filter/1(Out) -> Relay/1, Vdc/1
  "pole pairs "/1 -> Math Function/1
  rad_sens/1 -> "pole pairs "/1
  Math Function/1 -> theta/1
  iabc_sens/1 -> iabc/1
  pole pairs/1 -> Lowpass Filter/1, Scope/1
  Lowpass Filter/1 -> we/1, Scope/2

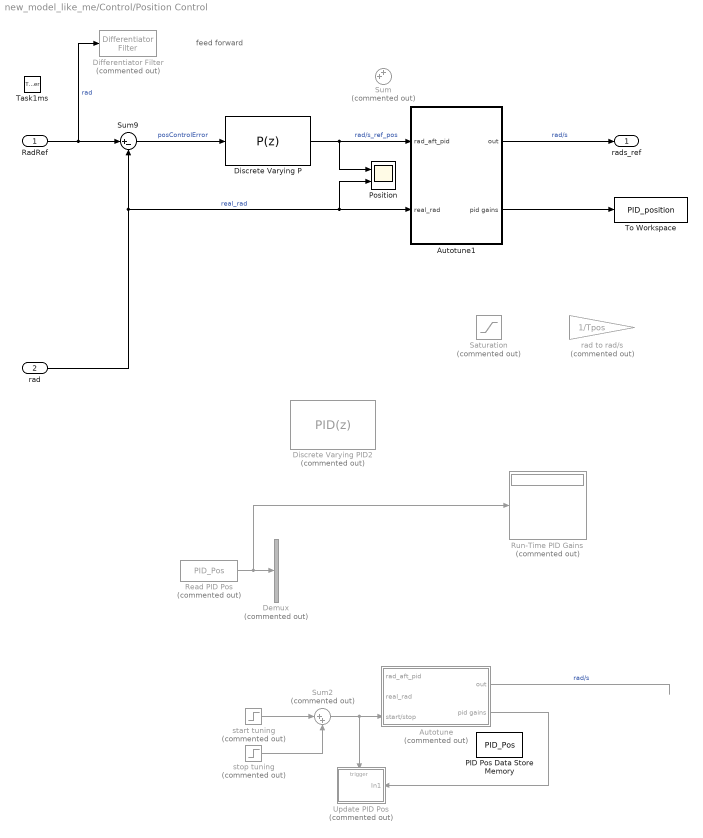
== system new_model_like_me/Control/Position Control ==
  note: feed forward
  RadRef : Inport
  rad : Inport  Port=2
  Task1ms : TriggerPort  TriggerType=function-call  VariantControl=Variant  PortDimensions=1
  Autotune : Subsystem  Commented=on
  Autotune1 : Subsystem
  Demux : Demux  Commented=on
  Differentiator Filter : dspfdesign/Differentiator Filter  Commented=on  DesignForMinimumOrder=on  FilterOrder=31  PassbandRipple=0.1  ScaleCoefficients=off  SimulateUsing=Interpreted execution  roundingMode=Floor  coeffsDataTypeStr=fixdt(1,16)
  Discrete Varying P : slpidlib/PID Controller  Controller=P  Form=Parallel  TimeDomain=Discrete-time  UseExternalTs=off  SampleTime=-1  IntegratorMethod=Forward Euler  FilterMethod=Forward Euler  ControllerParametersSource=internal  P=Kp_pos  I=Ki_pos  UseKiTs=off  D=Kd_pos  N=Kn_pos  UseFilter=on  TunerSelectOption=Transfer Function Based (PID Tuner App)  InitialConditionSource=internal  InitialConditionForIntegrator=0  InitialConditionForFilter=0  DifferentiatorICPrevScaledInput=0  ExternalReset=none  TrackingMode=on  Kt=1  LimitOutput=off  SatLimitsSource=internal  UpperSaturationLimit=LimA2up * pi/180  LowerSaturationLimit=LimA2down * pi/180  LinearizeAsGain=on  AntiWindupMode=none  Kb=1  LimitIntegrator=off  UpperIntegratorSaturationLimit=inf  LowerIntegratorSaturationLimit=-inf  POutMin=[]  POutMax=[]  IOutMin=[]  IOutMax=[]  DOutMin=[]  DOutMax=[]  NOutMin=[]  NOutMax=[]  SumOutMin=[]  SumOutMax=[]  SaturationOutMin=[]  SaturationOutMax=[]  PParamMin=[]  PParamMax=[]  IParamMin=[]  IParamMax=[]  DParamMin=[]  DParamMax=[]  NParamMin=[]  NParamMax=[]  KbParamMin=[]  KbParamMax=[]  KtParamMin=[]  KtParamMax=[]  KbOutMin=[]  KbOutMax=[]  KtOutMin=[]  KtOutMax=[]  IntegratorOutMin=[]  IntegratorOutMax=[]  FilterOutMin=[]  FilterOutMax=[]  SumI1OutMin=[]  SumI1OutMax=[]  SumI2OutMin=[]  SumI2OutMax=[]  SumI3OutMin=[]  SumI3OutMax=[]  SumI4OutMin=[]  SumI4OutMax=[]  SumDOutMin=[]  SumDOutMax=[]  DifferentiatorOutMin=[]  DifferentiatorOutMax=[]  FilterDiffOutCoefMin=[]  FilterDiffOutCoefMax=[]  ReciprocalOutMin=[]  ReciprocalOutMax=[]  SumDenOutMin=[]  SumDenOutMax=[]  SumNumOutMin=[]  SumNumOutMax=[]  DivideOutMin=[]  DivideOutMax=[]  UdiffTsProdOutMin=[]  UdiffTsProdOutMax=[]  NTsProdOutMin=[]  NTsProdOutMax=[]  UintegralTsProdOutMin=[]  UintegralTsProdOutMax=[]  UngainTsProdOutMin=[]  UngainTsProdOutMax=[]  ClampingZeroOutDataTypeStr=Inherit: Inherit via back propagation  ClampingZeroOutMin=[]  ClampingZeroOutMax=[]  FilterDenConstantOutDataTypeStr=Inherit: Inherit via back propagation  FilterDenConstantOutMin=[]  FilterDenConstantOutMax=[]  PCopyOutDataTypeStr=Inherit: Inherit via back propagation  PCopyOutMin=[]  PCopyOutMax=[]  NCopyOutDataTypeStr=Inherit: Inherit via back propagation  NCopyOutMin=[]  NCopyOutMax=[]  IntegratorContinuousStateAttributes=''  IntegratorStateMustResolveToSignalObject=off  IntegratorRTWStateStorageClass=Auto  FilterContinuousStateAttributes=''  FilterStateMustResolveToSignalObject=off  FilterRTWStateStorageClass=Auto  ParallelPVariant=InternalParameters  IdealPVariant=Disabled  IVariant=Disabled  DVariant=Disabled  IntegratorVariant=Disabled  SatVariant=Disabled  AWVariant=Disabled  PCopyVariant=Disabled  TRVariant=Disabled  FdbkBlocksVariant=Forward  IdealPFdbkVariant=Disabled  SatFdbkVariant=Disabled  DerivativeFilterVariant=Disabled  NVariant=Disabled  NCopyVariant=Disabled_SignalSpec  FilterICVariant=Disabled  IntegratorICVariant=Disabled  ExternalResetVariant=Disabled  TRSumVariant=Passthrough  SumFdbkVariant=Disabled  SumVariant=Passthrough_P  TsampFilterVariant=InternalTs  TsampNgainVariant=Passthrough  TsampIntegralVariant=Disabled_SignalSpec  ExternalSaturationOutDataTypeStr=Inherit: Same as second input
      settings: LibrarySourceBlock=cstblocks/Linear Parameter Varying/Discrete Varying PID
  Discrete Varying PID2 : slpidlib/PID Controller  Commented=on  Controller=PID  Form=Parallel  TimeDomain=Discrete-time  UseExternalTs=off  SampleTime=-1  IntegratorMethod=Forward Euler  FilterMethod=Forward Euler  ControllerParametersSource=internal  P=Kp_pos  I=Ki_pos  UseKiTs=off  D=Kd_pos  N=Kn_pos  UseFilter=on  TunerSelectOption=Transfer Function Based (PID Tuner App)  InitialConditionSource=internal  InitialConditionForIntegrator=0  InitialConditionForFilter=0  DifferentiatorICPrevScaledInput=0  ExternalReset=none  TrackingMode=on  Kt=1  LimitOutput=off  SatLimitsSource=internal  UpperSaturationLimit=LimA2up * pi/180  LowerSaturationLimit=LimA2down * pi/180  LinearizeAsGain=on  AntiWindupMode=none  Kb=1  LimitIntegrator=off  UpperIntegratorSaturationLimit=inf  LowerIntegratorSaturationLimit=-inf  POutMin=[]  POutMax=[]  IOutMin=[]  IOutMax=[]  DOutMin=[]  DOutMax=[]  NOutMin=[]  NOutMax=[]  SumOutMin=[]  SumOutMax=[]  SaturationOutMin=[]  SaturationOutMax=[]  PParamMin=[]  PParamMax=[]  IParamMin=[]  IParamMax=[]  DParamMin=[]  DParamMax=[]  NParamMin=[]  NParamMax=[]  KbParamMin=[]  KbParamMax=[]  KtParamMin=[]  KtParamMax=[]  KbOutMin=[]  KbOutMax=[]  KtOutMin=[]  KtOutMax=[]  IntegratorOutMin=[]  IntegratorOutMax=[]  FilterOutMin=[]  FilterOutMax=[]  SumI1OutMin=[]  SumI1OutMax=[]  SumI2OutMin=[]  SumI2OutMax=[]  SumI3OutMin=[]  SumI3OutMax=[]  SumI4OutMin=[]  SumI4OutMax=[]  SumDOutMin=[]  SumDOutMax=[]  DifferentiatorOutMin=[]  DifferentiatorOutMax=[]  FilterDiffOutCoefMin=[]  FilterDiffOutCoefMax=[]  ReciprocalOutMin=[]  ReciprocalOutMax=[]  SumDenOutMin=[]  SumDenOutMax=[]  SumNumOutMin=[]  SumNumOutMax=[]  DivideOutMin=[]  DivideOutMax=[]  UdiffTsProdOutMin=[]  UdiffTsProdOutMax=[]  NTsProdOutMin=[]  NTsProdOutMax=[]  UintegralTsProdOutMin=[]  UintegralTsProdOutMax=[]  UngainTsProdOutMin=[]  UngainTsProdOutMax=[]  ClampingZeroOutDataTypeStr=Inherit: Inherit via back propagation  ClampingZeroOutMin=[]  ClampingZeroOutMax=[]  FilterDenConstantOutDataTypeStr=Inherit: Inherit via back propagation  FilterDenConstantOutMin=[]  FilterDenConstantOutMax=[]  PCopyOutDataTypeStr=Inherit: Inherit via back propagation  PCopyOutMin=[]  PCopyOutMax=[]  NCopyOutDataTypeStr=Inherit: Inherit via back propagation  NCopyOutMin=[]  NCopyOutMax=[]  IntegratorContinuousStateAttributes=''  IntegratorStateMustResolveToSignalObject=off  IntegratorRTWStateStorageClass=Auto  FilterContinuousStateAttributes=''  FilterStateMustResolveToSignalObject=off  FilterRTWStateStorageClass=Auto  ParallelPVariant=InternalParameters  IdealPVariant=Disabled  IVariant=InternalParameters  DVariant=InternalParameters  IntegratorVariant=Discrete  SatVariant=Disabled  AWVariant=Passthrough  PCopyVariant=Disabled  TRVariant=Enabled  FdbkBlocksVariant=Forward  IdealPFdbkVariant=Disabled  SatFdbkVariant=Disabled  DerivativeFilterVariant=ForwardEulerFilter  NVariant=InternalParameters  NCopyVariant=Disabled  FilterICVariant=InternalICsFilter  IntegratorICVariant=InternalICs  ExternalResetVariant=Disabled  TRSumVariant=TrackingMode  SumFdbkVariant=Disabled  SumVariant=Sum_PID  TsampFilterVariant=InternalTs  TsampNgainVariant=Passthrough  TsampIntegralVariant=Disabled_SignalSpec  ExternalSaturationOutDataTypeStr=Inherit: Same as second input
      settings: LibrarySourceBlock=cstblocks/Linear Parameter Varying/Discrete Varying PID
  PID Pos Data Store Memory : DataStoreMemory  DataStoreName=PID_Pos  InitialValue=[Kp_pos 0 0 0]  ShowAdditionalParam=off
  Position : Scope  NumInputPorts=2
  Read PID Pos : DataStoreRead  Commented=on  DataStoreName=PID_Pos  IndexOptions=Index vector (dialog)  Indices=1  OutputSizes=1
  Run-Time PID Gains : Display  Commented=on
  Saturation : Saturate  Commented=on  UpperLimit=Wmax  LowerLimit=-Wmax
  Sum : Sum  Commented=on  Inputs=++|
  Sum2 : Sum  Commented=on  Inputs=|++
  Sum9 : Sum  Inputs=|+-
  To Workspace : ToWorkspace  VariableName=PID_position  SampleTime=-1
  Update PID Pos : Subsystem  Commented=on
  rad to rad/s : Gain  Commented=on  Gain=1/Tpos
  start tuning : Step  Commented=on  Time=Tpos_start
  stop tuning : Step  Commented=on  Time=Tpos_stop  After=-1
  rads_ref : Outport
  wires:
  rad/1 -> Sum9/2, Position/2, Autotune1/2(real_rad)  "real_rad"
  RadRef/1 -> Differentiator Filter/1, Sum9/1  "rad"
  Sum9/1 -> Discrete Varying P/1  "posControlError"
  stop tuning/1 -> Sum2/2
  start tuning/1 -> Sum2/1
  Sum2/1 -> Autotune/3(start/stop), Update PID Pos/Trigger
  Autotune/2(pid gains) -> Update PID Pos/1(In1)
  Autotune1/2(pid gains) -> To Workspace/1
  Autotune/1(out) -> ?  "rad/s"
  ? -> Autotune/2(real_rad)
  Read PID Pos/1 -> Run-Time PID Gains/1, Demux/1
  Discrete Varying P/1 -> Position/1, Autotune1/1(rad_aft_pid)  "rad/s_ref_pos"
  ? -> Sum/1
  Autotune1/1(out) -> rads_ref/1  "rad/s"
